simulink model "checkRadiation_in_WetherFromFile"  (Simulink 7.6)
settings: Solver=ode45  StartTime=90*24*3600  StopTime=100*24*3600  RelTol=1e-3
libraries: carnot x3
settings Model: Creator=drhf  LastModifiedBy=drhf
settings CodeAppCC: CustomSymbolStrType=$N$R$M_T

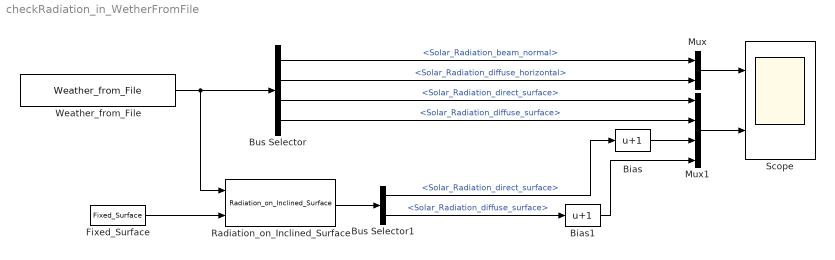
== system checkRadiation_in_WetherFromFile ==
  Bias : Bias  Bias=1
  Bias1 : Bias  Bias=1
  Bus Selector : BusSelector  OutputSignals=Solar_Radiation_beam_normal,Solar_Radiation_diffuse_horizontal,Solar_Radiation_direct_surface,Solar_Radiation_diffuse_surface
  Bus Selector1 : BusSelector  OutputSignals=Solar_Radiation_direct_surface,Solar_Radiation_diffuse_surface
  Fixed_Surface : carnot/Weather/Fixed_Surface  SystemSampleTime=-1  colangle=0  colazi=0  colrot=0
  Mux : Mux  Inputs=2
  Mux1 : Mux
  Radiation_on_Inclined_Surface : carnot/Weather/Radiation_on_Inclined_Surface  SystemSampleTime=-1  sky=Perez 1990  reflect=0.2
  Scope : Scope  NumInputPorts=2
      settings: YMin=-5~-5  YMax=5~5
  Weather_from_File : carnot/Weather/Weather_from_File  SystemSampleTime=-1  file=DE_TRY2010_02_averageYear  ext=.mat
  wires:
  Weather_from_File/1 -> Bus Selector/1, Radiation_on_Inclined_Surface/1
  Bus Selector/1 -> Mux/1  "<Solar_Radiation_beam_normal>"
  Bus Selector/2 -> Mux/2  "<Solar_Radiation_diffuse_horizontal>"
  Bus Selector/3 -> Mux1/1  "<Solar_Radiation_direct_surface>"
  Bus Selector/4 -> Mux1/2  "<Solar_Radiation_diffuse_surface>"
  Mux/1 -> Scope/1
  Mux1/1 -> Scope/2
  Fixed_Surface/1 -> Radiation_on_Inclined_Surface/2
  Bus Selector1/1 -> Bias/1  "<Solar_Radiation_direct_surface>"
  Bus Selector1/2 -> Bias1/1  "<Solar_Radiation_diffuse_surface>"
  Radiation_on_Inclined_Surface/1 -> Bus Selector1/1
  Bias/1 -> Mux1/3
  Bias1/1 -> Mux1/4
